simulink model "APPValuewithLookUpTable"  (R2023a)
settings: Solver=FixedStepDiscrete  StartTime=0.0  StopTime=10.0  FixedStep=0.005  RelTol=1e-3
undefined symbols (not defined in the file): TPSPercentBkpt, TPSPercentTbl, Ts
settings Model: Creator=The MathWorks, Inc.  LastModifiedBy=omert
settings SolverCC: AlgebraicLoopSolver=TrustRegion
settings DataIOCC: SaveFormat=StructureWithTime
settings OptimizationCC: DefaultParameterBehavior=Inlined  EnhancedBackFolding=on  PassReuseOutputArgsAs=Individual arguments  ZeroExternalMemoryAtStartup=off  ZeroInternalMemoryAtStartup=off  OptimizeBlockOrder=speed  DifferentSizesBufferReuse=on  OptimizationCustomize=off  EfficientTunableParamExpr=on
settings DebuggingCC: ParameterTunabilityLossMsg=error  UnconnectedInputMsg=warning  UnconnectedOutputMsg=warning  UnconnectedLineMsg=warning
settings ModelReferenceCC: EnableRefExpFcnMdlSchedulingChecks=on
settings SFSimCC: MATLABDynamicMemAlloc=off
settings RTWCC: Description=Embedded Coder  SystemTargetFile=ert.tlc  GenCodeOnly=on  TemplateMakefile=ert_default_tmf  DLArmComputeVersion=19.05
settings CodeAppCC: ForceParamTrailComments=on  IgnoreCustomStorageClasses=off  MaxIdLength=255  OperatorAnnotations=on  SimulinkDataObjDesc=on  SFDataObjDesc=on  InsertBlockDesc=on
settings ERTTargetCC: TargetLangStandard=C99 (ISO)  GenerateSampleERTMain=on  InlinedParameterPlacement=NonHierarchical  ERTCustomFileTemplate=example_file_process.tlc

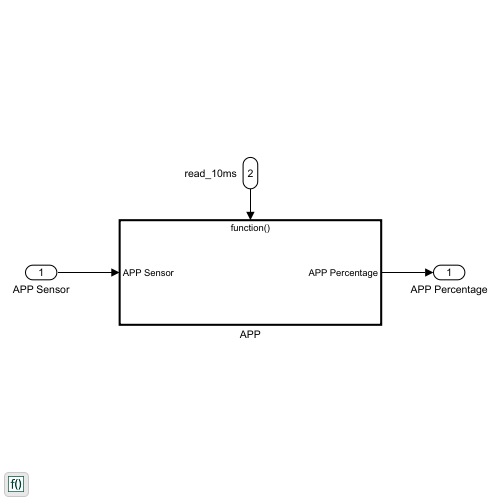
[thumbnail: Simulink's stored preview of the top-level diagram]
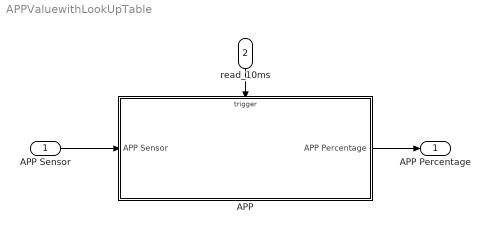
== system APPValuewithLookUpTable ==
  APP Sensor : Inport  OutDataTypeStr=uint16  PortDimensions=1
  read_10ms : Inport  Port=2  OutDataTypeStr=uint16  PortDimensions=1  SampleTime=0.02  OutputFunctionCall=on
  APP : Subsystem  TreatAsAtomicUnit=on  SystemSampleTime=0.005
  APP Percentage : Outport  OutDataTypeStr=single  PortDimensions=1
  wires:
  APP Sensor/1 -> APP/1(APP Sensor)
  APP/1(APP Percentage) -> APP Percentage/1
  read_10ms/1 -> APP/Trigger

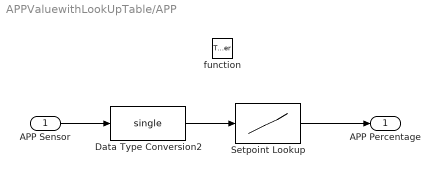
== system APPValuewithLookUpTable/APP ==
  APP Sensor : Inport
  function : TriggerPort  TriggerType=function-call  VariantControl=(inherit)  SampleTimeType=periodic  SampleTime=Ts*2  PortDimensions=1
  Data Type Conversion2 : DataTypeConversion  OutDataTypeStr=single  SaturateOnIntegerOverflow=off  RndMeth=Floor
  Setpoint Lookup : Lookup_n-D  NumberOfTableDimensions=1  DataSpecification=Lookup table object  LookupTableObject=Percent  BreakpointsForDimension1=TPSPercentBkpt  BreakpointsForDimension1DataTypeStr=single  IndexSearchMethod=Linear search  Table=TPSPercentTbl  TableDataTypeStr=single  ExtrapMethod=Clip  InternalRulePriority=Speed  OutDataTypeStr=single  RndMeth=Simplest
  APP Percentage : Outport
  wires:
  APP Sensor/1 -> Data Type Conversion2/1
  Setpoint Lookup/1 -> APP Percentage/1
  Data Type Conversion2/1 -> Setpoint Lookup/1
